simulink subsystem "Write_ULOG_Data"  (R2025a)
settings: Solver=VariableStepAuto  StartTime=0.0  StopTime=10.0  RelTol=1e-3
libraries: px4Utilslib x1
settings Model: Creator=gurt1  LastModifiedBy=gurt1
settings RTWCC: GPUComputeCapability=3.5

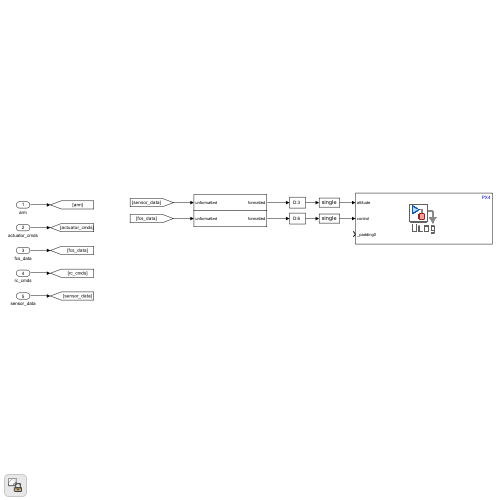
[thumbnail: Simulink's stored preview of the top-level diagram]
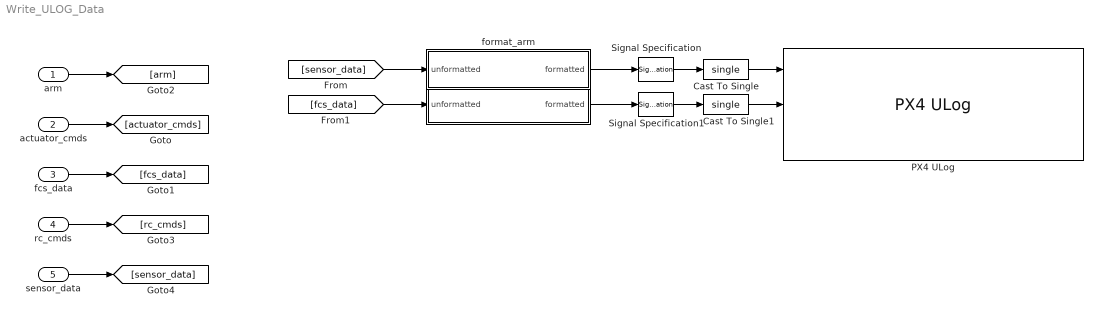
== system Write_ULOG_Data ==
  arm : Inport
  actuator_cmds : Inport  Port=2
  fcs_data : Inport  Port=3
  rc_cmds : Inport  Port=4
  sensor_data : Inport  Port=5
  " " : Subsystem
  Cast To Single : DataTypeConversion  OutDataTypeStr=single  SaturateOnIntegerOverflow=off  RndMeth=Floor
  Cast To Single1 : DataTypeConversion  OutDataTypeStr=single  SaturateOnIntegerOverflow=off  RndMeth=Floor
  PX4 ULog : px4Utilslib/PX4 ULog  uORBTopic=FcsSignals
  Signal Specification : SignalSpecification  Dimensions=3
  Signal Specification1 : SignalSpecification  Dimensions=6
  format_arm : Subsystem
  wires:
  actuator_cmds/1 -> [actuator_cmds]
  arm/1 -> [arm]
  fcs_data/1 -> [fcs_data]
  sensor_data/1 -> [sensor_data]
  rc_cmds/1 -> [rc_cmds]
  " "/1(formatted) -> Signal Specification1/1
  format_arm/1(formatted) -> Signal Specification/1
  [fcs_data] -> " "/1(unformatted)
  [sensor_data] -> format_arm/1(unformatted)
  Signal Specification/1 -> Cast To Single/1
  Signal Specification1/1 -> Cast To Single1/1
  Cast To Single/1 -> PX4 ULog/1
  Cast To Single1/1 -> PX4 ULog/2

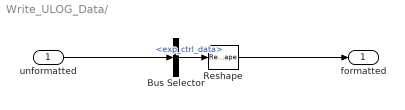
== system Write_ULOG_Data/  ==
  unformatted : Inport
  Bus Selector : BusSelector  OutputSignals=exp_ctrl_data
  Reshape : Reshape
  formatted : Outport
  wires:
  Bus Selector/1 -> Reshape/1  "<exp_ctrl_data>"
  Reshape/1 -> formatted/1
  unformatted/1 -> Bus Selector/1

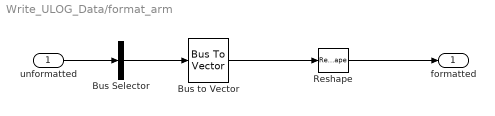
== system Write_ULOG_Data/format_arm ==
  unformatted : Inport
  Bus Selector : BusSelector  OutputSignals=att_rad  OutputAsBus=on
  Bus to Vector : BusToVector
  Reshape : Reshape
  formatted : Outport
  wires:
  Bus to Vector/1 -> Reshape/1
  unformatted/1 -> Bus Selector/1
  Reshape/1 -> formatted/1
  Bus Selector/1 -> Bus to Vector/1
